simulink model "power_hvdc12_fault"  (R2016a)
settings: Solver=FixedStepDiscrete  SolverMode=SingleTasking  StartTime=0.0  StopTime=2  FixedStep=Ts  RelTol=1e-3  AbsTol=1e-2
InitFcn:
  | Ts=50e-6;
  | 
  | % Rectifier AC side :
  | VLL_nom_R = 500e3; % V
  | Fnom_R = 60;           % Hz
  | 
  | % Inverter AC side :
  | VLL_nom_I = 345e3; % V
  | Fnom_I = 50;           % Hz
  | 
  | % DC :
  | Vdc_nom = 500e3;   % V
  | Idc_nom  = 2000;     % A
values from neighbouring files (symbols this model uses):
  m = mrand(i)    [01_Generate_TrainData_script.m]    (also in 05_Generate_TestData_script.m)
  MyTs = 1.0e-4    (= 0.0001)    [01_Generate_TrainData_script.m]    (also in 05_Generate_TestData_script.m)
undefined symbols (not defined in the file or in its folder): D1, Delta, lagging, pulse, test_alpha
libraries: powerlib_meascontrol x57, powerlib x43, simulink x24
(part 2 of 5)

== system power_hvdc12_fault/Inverter Control and Protection/Gamma Measurement ==
  Vabc : Inport
  I_th(1-6)_Y : Inport  Port=2
  I_th(1-6)_D : Inport  Port=3
  Freq : Inport  Port=4
  PulsesY : Inport  Port=5
  PulsesD : Inport  Port=6
  A--> pu : Gain  Gain=1/Idc_nom  SaturateOnIntegerOverflow=on  OutDataTypeStr=Inherit: Same as input  ParamDataTypeStr=Inherit: Same as input
  "A--> pu " : Gain  Gain=1/Idc_nom  SaturateOnIntegerOverflow=on  OutDataTypeStr=Inherit: Same as input  ParamDataTypeStr=Inherit: Same as input
  Gamma Measurement (D1 bridge) : Subsystem  DialogController=POWERSYS.PowerSysDialog  mask(Discrete Gamma Measurement (6-pulse converter)){transfo_type=Yg / D1(lag), f0=Fnom_I, Ith_min=0.001, Interpolation=on, V_tol=0.01, Ts=Ts}
      mask prompts: transfo_type "Transformer connection:"; f0 "Base frequency (Hz):"; Ith_min "Current threshold for thyristor zero-current detection (pu or A):"; Interpolation "Use interpolation"; V_tol "Voltage threshold for linear interpolation  (pu or V):"; Ts "Sample time (s):"
      mask help:
      | This block measures the extinction angle Gamma of a 6-pulse thyristor converter.
      |
      | Press Help for details.
      mask init:
      | powericon('psbcallbacks',gcb,'Discrete Gamma Measurement');
      | power_initmask();
      | if strcmp(Interpolation,'on')
      |     InterpolationOn=1;
      | else
      |     InterpolationOn=0;
      | end
      mask Help:
      | This block measures the extinction angle Gamma for each of the 6 thyristors
      | of a 6-pulse thyristor converter.
      | 
      | Gamma is the time expressed in degrees from the thyristor normal current
      | extinction to the time when the thyristor commutation voltage Vak becomes
      | positive. If interpolation is activated, Gamma is evaluated more precisely
      | by predicting the "exact" zero crossing instant of commutation voltage.
      | Interpolation is applied only if the voltage variation between the two
      | voltage samples on each side of zero-crossing exceeds the value specified
      | in the "Voltage threshold for interpolation" parameter (recommended value
      | 1% of nominal voltage).
      | 
      | The system frequency (input 3) is used to convert time values in electrical
      |  degrees. The current extinction time is determined from the "Current
      | threshold" parameter (recommended value 0.1% of nominal current). Valve
      | gate pulses (input 4) are used to discriminate between a current extinction
      |  during normal commutation sequence (valve gate pulse no longer present)
      | and premature extinction due to current discontinuity when DC current
      | reference Id_ref is low, (typically Id_ref<0.1 pu). If gate pulses are not
      | connected to input 4, Gamma measurement will stay correct as long as there
      | is no discontinuity in valve current pulses.
      | 
      | The 6 Gamma angles are determined using the 6 thyristor currents (input 1)
      | and the 6 commutation voltages derived from the three phase-to-ground AC
      | voltages measured at the primary of the converter transformer (input 2).
      | The secondary winding connection of the converter transformer (Y or Delta)
      | is selectable from the "Transformer connection" parameter. This information
      |  is important to derive the correct commutation voltage, for the outgoing
      | valve, from the primary voltages.
      | 
      | Output 1 = minimum value of the 6 Gamma angles over a rolling window of 6
      | consecutive extinctions; Output 2= mean value of the 6 Gamma angles; Output
      |  3 = vector of 6 commutation voltages used in the determination of Gamma,
      | assuming a 1:1 converter transformer ratio; Output 4= scalar output of the
      | six gamma angles.
      mask TypeOptions transfo_type: Yg / Y | Yg / D1(lag) | Yg / D11(lead)
      mask Callback Interpolation: powericon('psbcallbacks',gcb,'Discrete Gamma Measurement');
      mask Display: disp('\n\n\n')
  Gamma Measurement (Y bridge) : Subsystem  DialogController=POWERSYS.PowerSysDialog  mask(Discrete Gamma Measurement (6-pulse converter)){transfo_type=Yg / Y, f0=Fnom_I, Ith_min=0.001, Interpolation=on, V_tol=0.01, Ts=Ts}
      mask prompts: transfo_type "Transformer connection:"; f0 "Base frequency (Hz):"; Ith_min "Current threshold for thyristor zero-current detection (pu or A):"; Interpolation "Use interpolation"; V_tol "Voltage threshold for linear interpolation  (pu or V):"; Ts "Sample time (s):"
      mask help:
      | This block measures the extinction angle Gamma of a 6-pulse thyristor converter.
      |
      | Press Help for details.
      mask init:
      | powericon('psbcallbacks',gcb,'Discrete Gamma Measurement');
      | power_initmask();
      | if strcmp(Interpolation,'on')
      |     InterpolationOn=1;
      | else
      |     InterpolationOn=0;
      | end
      mask Help:
      | This block measures the extinction angle Gamma for each of the 6 thyristors
      | of a 6-pulse thyristor converter.
      | 
      | Gamma is the time expressed in degrees from the thyristor normal current
      | extinction to the time when the thyristor commutation voltage Vak becomes
      | positive. If interpolation is activated, Gamma is evaluated more precisely
      | by predicting the "exact" zero crossing instant of commutation voltage.
      | Interpolation is applied only if the voltage variation between the two
      | voltage samples on each side of zero-crossing exceeds the value specified
      | in the "Voltage threshold for interpolation" parameter (recommended value
      | 1% of nominal voltage).
      | 
      | The system frequency (input 3) is used to convert time values in electrical
      |  degrees. The current extinction time is determined from the "Current
      | threshold" parameter (recommended value 0.1% of nominal current). Valve
      | gate pulses (input 4) are used to discriminate between a current extinction
      |  during normal commutation sequence (valve gate pulse no longer present)
      | and premature extinction due to current discontinuity when DC current
      | reference Id_ref is low, (typically Id_ref<0.1 pu). If gate pulses are not
      | connected to input 4, Gamma measurement will stay correct as long as there
      | is no discontinuity in valve current pulses.
      | 
      | The 6 Gamma angles are determined using the 6 thyristor currents (input 1)
      | and the 6 commutation voltages derived from the three phase-to-ground AC
      | voltages measured at the primary of the converter transformer (input 2).
      | The secondary winding connection of the converter transformer (Y or Delta)
      | is selectable from the "Transformer connection" parameter. This information
      |  is important to derive the correct commutation voltage, for the outgoing
      | valve, from the primary voltages.
      | 
      | Output 1 = minimum value of the 6 Gamma angles over a rolling window of 6
      | consecutive extinctions; Output 2= mean value of the 6 Gamma angles; Output
      |  3 = vector of 6 commutation voltages used in the determination of Gamma,
      | assuming a 1:1 converter transformer ratio; Output 4= scalar output of the
      | six gamma angles.
      mask TypeOptions transfo_type: Yg / Y | Yg / D1(lag) | Yg / D11(lead)
      mask Callback Interpolation: powericon('psbcallbacks',gcb,'Discrete Gamma Measurement');
      mask Display: disp('\n\n\n')
  MinMax1 : MinMax  Inputs=2  SaturateOnIntegerOverflow=on  InputSameDT=on
  Selector : Selector  InputPortWidth=6  IndexOptions=Index vector (dialog)  Indices=1  OutputSizes=1
  Selector1 : Selector  InputPortWidth=6  IndexOptions=Index vector (dialog)  Indices=1  OutputSizes=1
  Sum1 : Sum  SaturateOnIntegerOverflow=on  InputSameDT=on  OutDataTypeStr=Inherit: Same as first input
  Terminator1 : Terminator
  Terminator2 : Terminator
  Terminator3 : Terminator
  k : Gain  Gain=0.5  SaturateOnIntegerOverflow=on  OutDataTypeStr=Inherit: Same as input  ParamDataTypeStr=Inherit: Same as input
  gamma_min : Outport
  gamma_mean : Outport  Port=2
  tag scope: ISw1Y_pu=global, Ucom1Y_pu=global
  wires:
  I_th(1-6)_Y/1 -> A--> pu/1
  A--> pu/1 -> Gamma Measurement (Y bridge)/1(I_th(1-6)), Selector1/1
  Vabc/1 -> Gamma Measurement (D1 bridge)/2(Uabc), Gamma Measurement (Y bridge)/2(Uabc)
  Gamma Measurement (Y bridge)/1(gamma_min (deg)) -> MinMax1/1  "gamma min Y"
  Gamma Measurement (Y bridge)/3(Ucom(1-6)) -> Selector/1
  Gamma Measurement (Y bridge)/2(gamma_mean (deg)) -> Sum1/1
  I_th(1-6)_D/1 -> "A--> pu "/1
  "A--> pu "/1 -> Gamma Measurement (D1 bridge)/1(I_th(1-6))
  Gamma Measurement (D1 bridge)/3(Ucom(1-6)) -> Terminator2/1
  Gamma Measurement (D1 bridge)/2(gamma_mean (deg)) -> Sum1/2
  Gamma Measurement (D1 bridge)/1(gamma_min (deg)) -> MinMax1/2  "gamma min D"
  MinMax1/1 -> gamma_min/1
  Sum1/1 -> k/1
  k/1 -> gamma_mean/1
  Selector/1 -> [Ucom1Y_pu]
  Selector1/1 -> [ISw1Y_pu]
  Freq/1 -> Gamma Measurement (D1 bridge)/3(Freq), Gamma Measurement (Y bridge)/3(Freq)
  Gamma Measurement (D1 bridge)/4(gamma (deg)) -> Terminator1/1
  Gamma Measurement (Y bridge)/4(gamma (deg)) -> Terminator3/1
  PulsesY/1 -> Gamma Measurement (Y bridge)/4(Pulses(1-6))
  PulsesD/1 -> Gamma Measurement (D1 bridge)/4(Pulses(1-6))

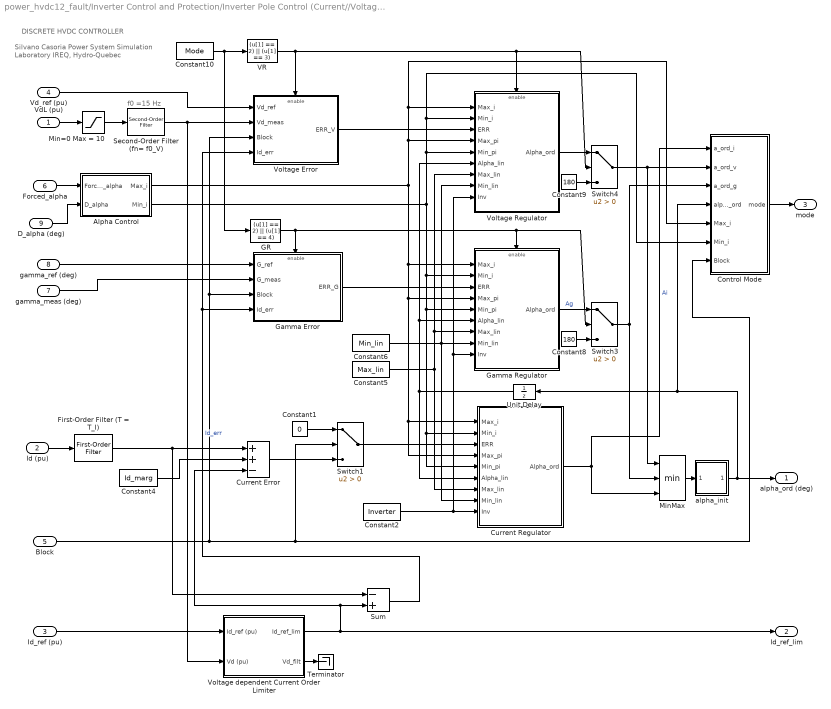
== system power_hvdc12_fault/Inverter Control and Protection/Inverter Pole Control (Current//Voltage//Gamma) ==
  note: DISCRETE HVDC CONTROLLER
  note: Silvano Casoria
      | Power System Simulation Laboratory
      |  IREQ, Hydro-Quebec
  note: f0 =15 Hz
  VdL (pu) : Inport
  Id (pu) : Inport  Port=2
  Id_ref (pu) : Inport  Port=3
  Vd_ref (pu) : Inport  Port=4
  Block : Inport  Port=5
  Forced_alpha : Inport  Port=6
  gamma_meas (deg) : Inport  Port=7
  gamma_ref (deg) : Inport  Port=8
  D_alpha (deg) : Inport  Port=9
  Alpha Control : Subsystem
  Constant1 : Constant  Value=0
  Constant10 : Constant  Value=Mode
  Constant2 : Constant  Value=Inverter
  Constant4 : Constant  Value=Id_marg
  Constant5 : Constant  Value=Max_lin
  Constant6 : Constant  Value=Min_lin
  Constant8 : Constant  Value=180
  Constant9 : Constant  Value=180
  "Control Mode " : Subsystem
  Current Error : Sum  Inputs=++-  SaturateOnIntegerOverflow=on  InputSameDT=on  OutDataTypeStr=Inherit: Same as first input
  Current Regulator : Subsystem  TreatAsAtomicUnit=on
  First-Order Filter (T = T_I) : powerlib_meascontrol/Filters/First-Order Filter  FilterType=Lowpass  Tc=T_I  Ts=Ts  Initialize=off  Vac_Init=[0, 0, 60]  Vdc_Init=0  PlotResponse=off  FreqRange="[0,  200,  1]"
  GR : Fcn  Expr=(u[1] == 2) || (u[1] == 4)
  Gamma Error : Subsystem  TreatAsAtomicUnit=on
  Gamma Regulator : Subsystem  TreatAsAtomicUnit=on
  Min=0 Max = 10 : Saturate  UpperLimit=10  LowerLimit=0
  MinMax : MinMax  Inputs=3  SaturateOnIntegerOverflow=on  InputSameDT=on
  Second-Order Filter (fn= f0_V) : powerlib_meascontrol/Filters/Second-Order Filter  FilterType=Lowpass  Fo=f0_V  Zeta=Z_V  Ts=Ts  Initialize=off  Vac_Init="[0,  0,  60]"  Vdc_Init=0  PlotResponse=off  FreqRange=[0, 500, 1]
  Sum : Sum  Inputs=-+  SaturateOnIntegerOverflow=on  InputSameDT=on  OutDataTypeStr=Inherit: Same as first input
  Switch1 : Switch  Criteria=u2 > Threshold  SaturateOnIntegerOverflow=on  InputSameDT=on
  Switch3 : Switch  Criteria=u2 > Threshold  SaturateOnIntegerOverflow=on  InputSameDT=on
  Switch4 : Switch  Criteria=u2 > Threshold  SaturateOnIntegerOverflow=on  InputSameDT=on
  Terminator : Terminator
  Unit Delay : UnitDelay  SampleTime=Ts
  VR : Fcn  Expr=(u[1] == 2) || (u[1] == 3)
  Voltage Error : Subsystem  TreatAsAtomicUnit=on
  Voltage Regulator : Subsystem  TreatAsAtomicUnit=on
  Voltage dependent Current Order Limiter : Subsystem  mask(Voltage Dependent Current Order Limiter  (Discrete)){Vd_seuil=Vd_seuil, Vd_min=Vd_min, Id_min=Id_min, Id_min_abs=Id_min_abs, Tu=Tup, Ts=Ts}
      mask prompts: Vd_seuil "Vd seuil (pu):"; Vd_min "Vd min (pu):"; Id_min "Id min (pu):"; Id_min_abs "Id min abs (pu):"; Tu "Up Time constant (s):"; Ts "Sample time (s):"
      mask Display: disp('VDCOL\n (Discrete)')
  alpha_init : Subsystem
  alpha_ord (deg) : Outport
  Id_ref_lim : Outport  Port=2
  mode : Outport  Port=3
  wires:
  Voltage Regulator/1(Alpha_ord) -> Switch4/1
  GR/1 -> Gamma Error/Enable, Gamma Regulator/Enable, Switch3/2
  Constant10/1 -> VR/1, GR/1
  VR/1 -> Voltage Error/Enable, Switch4/2, Voltage Regulator/Enable
  D_alpha (deg)/1 -> Alpha Control/2(D_alpha)
  Alpha Control/1(Max_i) -> Current Regulator/1(Max_i), Current Regulator/4(Max_pi), Gamma Regulator/4(Max_pi), Gamma Regulator/1(Max_i), "Control Mode "/5(Max_i), Voltage Regulator/1(Max_i), Voltage Regulator/4(Max_pi)
  Constant6/1 -> Voltage Regulator/8(Min_lin), Gamma Regulator/8(Min_lin), Current Regulator/8(Min_lin)
  Constant4/1 -> Current Error/2
  Id_ref (pu)/1 -> Voltage dependent Current Order Limiter/1(Id_ref (pu))
  Voltage dependent Current Order Limiter/2(Vd_filt) -> Terminator/1
  Voltage dependent Current Order Limiter/1(Id_ref_lim) -> Id_ref_lim/1, Sum/2, Current Error/3
  Second-Order Filter (fn= f0_V)/1 -> Voltage dependent Current Order Limiter/2(Vd (pu)), Voltage Error/2(Vd_meas)
  Min=0 Max = 10/1 -> Second-Order Filter (fn= f0_V)/1
  VdL (pu)/1 -> Min=0 Max = 10/1
  Id (pu)/1 -> First-Order Filter (T = T_I)/1
  First-Order Filter (T = T_I)/1 -> Sum/1, Current Error/1
  Current Error/1 -> Switch1/3
  MinMax/1 -> alpha_init/1(In1)
  Unit Delay/1 -> Voltage Regulator/6(Alpha_lin), Gamma Regulator/6(Alpha_lin), Current Regulator/6(Alpha_lin)
  alpha_init/1(Out1) -> alpha_ord (deg)/1, Unit Delay/1, "Control Mode "/4(alpha_ord)
  Constant5/1 -> Voltage Regulator/7(Max_lin), Gamma Regulator/7(Max_lin), Current Regulator/7(Max_lin)
  Alpha Control/2(Min_i) -> Current Regulator/5(Min_pi), Current Regulator/2(Min_i), Gamma Regulator/5(Min_pi), Gamma Regulator/2(Min_i), "Control Mode "/6(Min_i), Voltage Regulator/2(Min_i), Voltage Regulator/5(Min_pi)
  Block/1 -> Switch1/2, "Control Mode "/7(Block), Gamma Error/3(Block), Voltage Error/3(Block)
  Constant2/1 -> Voltage Regulator/9(Inv), Gamma Regulator/9(Inv), Current Regulator/9(Inv)
  Switch1/1 -> Current Regulator/3(ERR)
  Gamma Regulator/1(Alpha_ord) -> Switch3/1  "Ag"
  Constant8/1 -> Switch3/3
  Constant9/1 -> Switch4/3
  Current Regulator/1(Alpha_ord) -> MinMax/3, "Control Mode "/1("a_ord_i ")  "Ai"
  Switch3/1 -> MinMax/2, "Control Mode "/3(a_ord_g)
  Switch4/1 -> MinMax/1, "Control Mode "/2(a_ord_v)
  Constant1/1 -> Switch1/1
  Gamma Error/1(ERR_G) -> Gamma Regulator/3(ERR)
  gamma_ref (deg)/1 -> Gamma Error/1(G_ref)
  gamma_meas (deg)/1 -> Gamma Error/2(G_meas)
  Sum/1 -> Voltage Error/4(Id_err), Gamma Error/4(Id_err)  "Id_err"
  Vd_ref (pu)/1 -> Voltage Error/1(Vd_ref)
  Voltage Error/1(ERR_V) -> Voltage Regulator/3(ERR)
  "Control Mode "/1(mode) -> mode/1
  Forced_alpha/1 -> Alpha Control/1(Forced_alpha)

== system power_hvdc12_fault/Inverter Control and Protection/Inverter Protections ==
  Uabc (pu) : Inport
  Commutation Failure Prevention Control (CFPREV) : Subsystem  mask(Commutation Failure Prevention Control){STATE=on, T_ss=0.64, ab_level=0.1, ab_gain=25, z_level=0.1, z_gain=25, fn=60, Filter=[2.0, 1.0], Ts=Ts}
      mask prompts: STATE "ON State"; T_ss "Simulation Steady_State Time (s):"; ab_level "ab level (pu):"; ab_gain "ab gain (deg/pu):"; z_level "z level (pu):"; z_gain "z gain (deg/pu):"; fn "Base frequency (Hz):"; Filter "Filter Time const. and Iinitial condition [T(s), Ic (pu)]:"; Ts "Sample Time (s):"
      mask help:
      | The protective function, used in the inverter, mitigates commutation failures due to AC voltage dips. After a fault detection (three-phase or one-phase) an angle value (AMIN_CFPREV) is sent to the converter control in order to be deducted from the maximum delay angle limit (alpha_max). Practically, the commutation margin is consequently enlarged reducing therefore the risk of commutation failures.
      |
      |      The CLARK transformation is used for three-phase fault  detection and the zero-sequence voltage evaluation. The detection is based  on instantaneous values, which ensure fast reaction of the control system when AC faults occurs.
      |
      |      Press Help to get the reference with the  detailed description of the function and  parameters.
      |
      | Note: To accelerate the function initialisation, the first parameter (Simulation Steady_State Time) is used. It corresponds to the time when the input voltages reache  the steady-state value.
      mask init:
      | T_periode = 0.6/fn;    % More then half the period
      | filt_tc = Filter(1);
      | filt_ic = Filter(2);
      | 
      | if (STATE)
      | 	str = 'ON';
      | else
      | 	str = 'OFF';
      | end
      mask Help:
      | Ref. "A Novel Method to Mitigate Commutation Failures in HVDC Systems,"
      | Lidong Zhang, Lars Dofnas ABB Utilities Power System Technology,
      | Proceedings PowerCon 2002, Volume: 1 , 13-17 Oct. 2002,  Page(s): 51-56 vol.1.
      mask Display: disp(['\n\n\n State:[',str,']'])
  First-Order Filter (T= 3.3 ms) : powerlib_meascontrol/Filters/First-Order Filter  FilterType=Lowpass  Tc=0.0033  Ts=Ts  Initialize=off  Vac_Init=[0, 0, 60]  Vdc_Init=0  PlotResponse=off  FreqRange="[0,  200,  1]"
  Informations : Subsystem
      mask Display: disp('?')
  Low  AC Voltage Detection (LACVD) : Subsystem  TreatAsAtomicUnit=on  mask(Low AC voltage detection){STATE=on, Ref_1=0.75, Ts=fix(0.001/Ts)*Ts}
      mask prompts: STATE "ON State"; Ref_1 "Detection level (pu):"; Ts "Sample time (s):"
      mask help:
      | This bloc detects a low AC voltage condition on the commutation busbar and is used in the DC protection scheme. Its purpose is to descriminate between a drop in the AC voltage caused by a fault on the DC line or by a fault on the AC side.
      |
      |      An AC fault detection (Low_ac_voltage output signal) will occur when the AC voltage input (recified three-phase AC voltage) drops below a certain reference value (Detection level).
      |
      |      In order to minimize the simulation time, an enabled susbystem having a sample time of 1 (ms) has been used in accordance with an acceptable precision.
      mask init:
      | if (STATE)
      | 	str = 'ON';
      | else
      | 	str = 'OFF';
      | end
      mask Display: disp(['\n\n\n\nState:[',str,']'])
  T = 1 ms : DiscretePulseGenerator  Period=fix(0.001/Ts)  SampleTime=Ts
  Udio_6p : Subsystem
  Low_AC_Voltage : Outport
  AMIN_CFPREV : Outport  Port=2
  wires:
  Uabc (pu)/1 -> Udio_6p/1(Uabc (pu)), Commutation Failure Prevention Control (CFPREV)/1(Uabc (pu))
  Low  AC Voltage Detection (LACVD)/1(Low_AC_Voltage) -> Low_AC_Voltage/1
  Commutation Failure Prevention Control (CFPREV)/1(AMIN_CFPREV (deg)) -> AMIN_CFPREV/1
  T = 1 ms/1 -> Low  AC Voltage Detection (LACVD)/Enable
  Udio_6p/1(Udio_6p) -> First-Order Filter (T= 3.3 ms)/1
  First-Order Filter (T= 3.3 ms)/1 -> Low  AC Voltage Detection (LACVD)/1(Uac (pu))

== system power_hvdc12_fault/Master Control/Informations ==
  note: For testing purpose,  a step can be activated and added to the reference current at both
      | converters.
  note: Master Control
  note: INTRODUCTION
  note: The rectifier and inverter current reference are generated in the master control. The reference
      | should be equal in both converters to avoid the loss of the margin. The converter starting and stopping is
      | initiated and the current reference can be ramped up or down.  A current step can be added to the
      | current reference for testing purpose.
  note: DESCRIPTION
  note: At start-up, both converters are deblocked and ramped up to the minimum current allowed in steady-state
      | with an adjustable rate  and application time in the "Start/Stop & Ramping Unit" subsystem. After the
      | system stabilisation the current is ramped up to its final value  with an adjustable rate and execution time.
      | Before stopping the converters the current is ramped down to the minimum reference.

== system power_hvdc12_fault/Master Control/Start//Stop ==
  note: Start/Stop sequence
  note: Start/Stop & Ramping
  note: Ramping
  Bistable : powerlib_meascontrol/Logic/Bistable  Qpriority=Set  ic=0  Ts=Ts
  Edge Detector_1 : powerlib_meascontrol/Logic/Edge Detector  model=Rising  ic=0  Ts=Ts
  Edge Detector_2 : powerlib_meascontrol/Logic/Edge Detector  model=Rising  ic=0  Ts=Ts
  Logical Operator3 : Logic  AllPortsSameDT=off
  Minimum ref : Constant  Value=Min_ref
  Relational Operator1 : RelationalOperator  Operator=<=
  S1 : Subsystem  mask(RAMPING UNIT){Min_ref=Min_ref, SS_ramp=SS_ramp, F_up=F_up, up_slope=up_slope, T_up=T_up, F_down=F_down, down_slope=down_slope, T_down=T_down}
      mask prompts: Min_ref "Minimum Value (pu):"; SS_ramp "Start-Stop ramp (pu/s):"; F_up "Final Up Value (pu):"; up_slope "Up Slope (pu/s):"; T_up "Ramping Up Time (s):"; F_down "Final Down Value (pu):"; down_slope "Down Slope (pu/s):"; T_down "Ramping Down Time (s):"
      mask init:
      | T_up_final      =  T_up + (F_up - Min_ref)/up_slope;
      | T_down_final =   T_down + (F_down-F_up)/down_slope;
      | T_ramp  = [0, T_up, T_up_final,  T_down,  T_down_final, 9999]';
      | U_ramp = [0, 0, F_up-Min_ref,  F_up-Min_ref,  F_down- Min_ref,  F_down - Min_ref]';
      mask Display: disp('Ramping\n Unit')
  Start (T_start) : Step  Time=T_start  SampleTime=Ts
  Stop (T_stop) : Step  Time=T_stop  SampleTime=Ts
  Unit Delay : UnitDelay  SampleTime=Ts
  Id_ref_ramp : Outport
  "Stop " : Outport  Port=2
  wires:
  S1/1(Out1) -> Unit Delay/1, Id_ref_ramp/1
  Minimum ref/1 -> Relational Operator1/2
  Unit Delay/1 -> Relational Operator1/1
  Start (T_start)/1 -> Edge Detector_1/1
  Bistable/1 -> S1/1(Start)  "Start"
  Relational Operator1/1 -> Logical Operator3/1
  Stop (T_stop)/1 -> Logical Operator3/2
  Logical Operator3/1 -> Edge Detector_2/1
  Bistable/2 -> "Stop "/1
  Edge Detector_1/1 -> Bistable/1
  Edge Detector_2/1 -> Bistable/2

== system power_hvdc12_fault/Rectifier/Rectifier ==
  Py : Inport
  Pd : Inport  Port=2
  Bridge D : powerlib/Power Electronics/Universal Bridge  Arms=3  SnubberResistance=2000  SnubberCapacitance=0.1e-6  Device=Thyristors  Ron=1e-3  Lon=0  ForwardVoltages="[  0.8  0.8  ]"  ForwardVoltage=0  GTOparameters=[ 10e-6 , 20e-6 ]  IGBTparameters=[ 1e-6 , 2e-6 ]  Measurements=None  Measurements_2=None  converterType=Rectifier
  Bridge Y : powerlib/Power Electronics/Universal Bridge  Arms=3  SnubberResistance=2000  SnubberCapacitance=0.1e-6  Device=Thyristors  Ron=1e-3  Lon=0  ForwardVoltages="[  0.8  0.8  ]"  ForwardVoltage=0  GTOparameters=[ 10e-6 , 20e-6 ]  IGBTparameters=[ 1e-6 , 2e-6 ]  Measurements=All voltages and currents  Measurements_2=None  converterType=Rectifier
  Ay : PMIOPort  Port=1  Side=Left
  By : PMIOPort  Port=2  Side=Left
  Cy : PMIOPort  Port=3  Side=Left
  Ad : PMIOPort  Port=4  Side=Left
  Bd : PMIOPort  Port=5  Side=Left
  Cd : PMIOPort  Port=6  Side=Left
  pos : PMIOPort  Port=7  Side=Right
  neg : PMIOPort  Port=8  Side=Right
  wires:
  Pd/1 -> Bridge D/1
  Py/1 -> Bridge Y/1
  connections:
  Bridge D/RConn2 -- neg/RConn1
  Cd/RConn1 -- Bridge D/LConn3
  Bd/RConn1 -- Bridge D/LConn2
  Ad/RConn1 -- Bridge D/LConn1
  Cy/RConn1 -- Bridge Y/LConn3
  By/RConn1 -- Bridge Y/LConn2
  Bridge Y/RConn1 -- pos/RConn1
  Ay/RConn1 -- Bridge Y/LConn1
  Bridge D/RConn1 -- Bridge Y/RConn2

== system power_hvdc12_fault/Rectifier Control and Protection/12-pulse Firing Control ==
  alpha_ord (deg) : Inport
  Vabc (pu) : Inport  Port=2
  Block : Inport  Port=3
  PLL (3ph) : powerlib_meascontrol/PLL/PLL (3ph)  Fmin=0.75 * PLL_f0  Par_Init="[PLL_ph  PLL_f0]"  ParK="[PLL_Kp  PLL_Ki  0]"  TcD=1e-4  MaxRateChangeFreq=12  FilterCutOffFreq=25  Ts=Ts  AGC=off
  "Pulse Generator (Thyristor, 12-Pulse)" : powerlib_meascontrol/Pulse & Signal Generators/Pulse Generator (Thyristor, 12-Pulse)  GenType=12-pulse  Delta=D1 (lagging)  pwidth=Pw  Double_Pulse=off  Ts=Ts
  PulsesY : Outport
  PulsesD : Outport  Port=2
  Freq : Outport  Port=3
  wires:
  Vabc (pu)/1 -> PLL (3ph)/1
  PLL (3ph)/2 -> "Pulse Generator (Thyristor, 12-Pulse)"/2
  alpha_ord (deg)/1 -> "Pulse Generator (Thyristor, 12-Pulse)"/1
  "Pulse Generator (Thyristor, 12-Pulse)"/1 -> PulsesY/1
  "Pulse Generator (Thyristor, 12-Pulse)"/2 -> PulsesD/1
  PLL (3ph)/1 -> Freq/1
  Block/1 -> "Pulse Generator (Thyristor, 12-Pulse)"/3

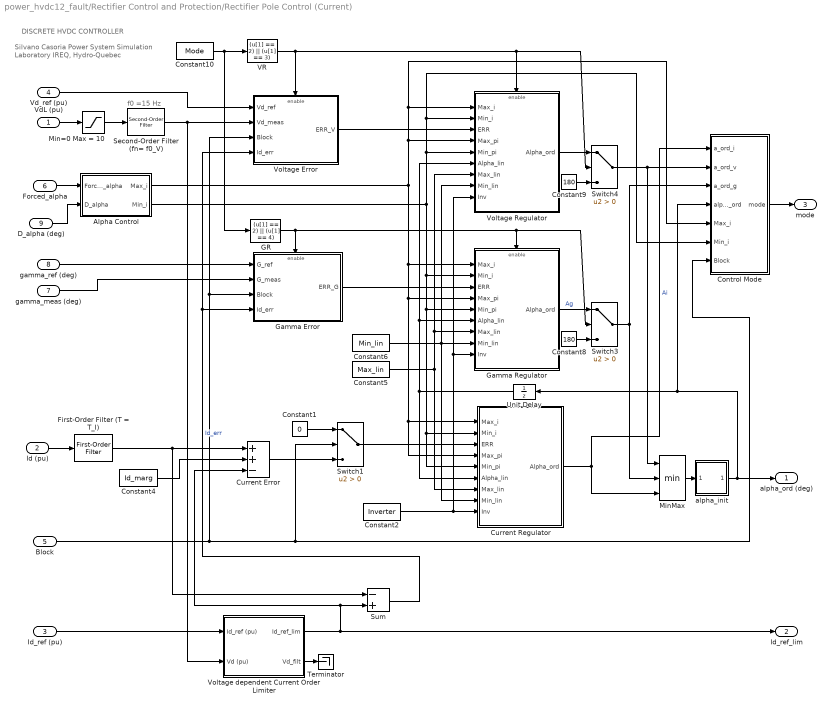
== system power_hvdc12_fault/Rectifier Control and Protection/Rectifier Pole Control (Current) ==
  note: DISCRETE HVDC CONTROLLER
  note: Silvano Casoria
      | Power System Simulation Laboratory
      |  IREQ, Hydro-Quebec
  note: f0 =15 Hz
  VdL (pu) : Inport
  Id (pu) : Inport  Port=2
  Id_ref (pu) : Inport  Port=3
  Vd_ref (pu) : Inport  Port=4
  Block : Inport  Port=5
  Forced_alpha : Inport  Port=6
  gamma_meas (deg) : Inport  Port=7
  gamma_ref (deg) : Inport  Port=8
  D_alpha (deg) : Inport  Port=9
  Alpha Control : Subsystem
  Constant1 : Constant  Value=0
  Constant10 : Constant  Value=Mode
  Constant2 : Constant  Value=Inverter
  Constant4 : Constant  Value=Id_marg
  Constant5 : Constant  Value=Max_lin
  Constant6 : Constant  Value=Min_lin
  Constant8 : Constant  Value=180
  Constant9 : Constant  Value=180
  "Control Mode " : Subsystem
  Current Error : Sum  Inputs=++-  SaturateOnIntegerOverflow=on  InputSameDT=on  OutDataTypeStr=Inherit: Same as first input
  Current Regulator : Subsystem  TreatAsAtomicUnit=on
  First-Order Filter (T = T_I) : powerlib_meascontrol/Filters/First-Order Filter  FilterType=Lowpass  Tc=T_I  Ts=Ts  Initialize=off  Vac_Init=[0, 0, 60]  Vdc_Init=0  PlotResponse=off  FreqRange="[0,  200,  1]"
  GR : Fcn  Expr=(u[1] == 2) || (u[1] == 4)
  Gamma Error : Subsystem  TreatAsAtomicUnit=on
  Gamma Regulator : Subsystem  TreatAsAtomicUnit=on
  Min=0 Max = 10 : Saturate  UpperLimit=10  LowerLimit=0
  MinMax : MinMax  Inputs=3  SaturateOnIntegerOverflow=on  InputSameDT=on
  Second-Order Filter (fn= f0_V) : powerlib_meascontrol/Filters/Second-Order Filter  FilterType=Lowpass  Fo=f0_V  Zeta=Z_V  Ts=Ts  Initialize=off  Vac_Init="[0,  0,  60]"  Vdc_Init=0  PlotResponse=off  FreqRange=[0, 500, 1]
  Sum : Sum  Inputs=-+  SaturateOnIntegerOverflow=on  InputSameDT=on  OutDataTypeStr=Inherit: Same as first input
  Switch1 : Switch  Criteria=u2 > Threshold  SaturateOnIntegerOverflow=on  InputSameDT=on
  Switch3 : Switch  Criteria=u2 > Threshold  SaturateOnIntegerOverflow=on  InputSameDT=on
  Switch4 : Switch  Criteria=u2 > Threshold  SaturateOnIntegerOverflow=on  InputSameDT=on
  Terminator : Terminator
  Unit Delay : UnitDelay  SampleTime=Ts
  VR : Fcn  Expr=(u[1] == 2) || (u[1] == 3)
  Voltage Error : Subsystem  TreatAsAtomicUnit=on
  Voltage Regulator : Subsystem  TreatAsAtomicUnit=on
  Voltage dependent Current Order Limiter : Subsystem  mask(Voltage Dependent Current Order Limiter  (Discrete)){Vd_seuil=Vd_seuil, Vd_min=Vd_min, Id_min=Id_min, Id_min_abs=Id_min_abs, Tu=Tup, Ts=Ts}
      mask prompts: Vd_seuil "Vd seuil (pu):"; Vd_min "Vd min (pu):"; Id_min "Id min (pu):"; Id_min_abs "Id min abs (pu):"; Tu "Up Time constant (s):"; Ts "Sample time (s):"
      mask Display: disp('VDCOL\n (Discrete)')
  alpha_init : Subsystem
  alpha_ord (deg) : Outport
  Id_ref_lim : Outport  Port=2
  mode : Outport  Port=3
  wires:
  Voltage Regulator/1(Alpha_ord) -> Switch4/1
  GR/1 -> Gamma Error/Enable, Gamma Regulator/Enable, Switch3/2
  Constant10/1 -> VR/1, GR/1
  VR/1 -> Voltage Error/Enable, Switch4/2, Voltage Regulator/Enable
  D_alpha (deg)/1 -> Alpha Control/2(D_alpha)
  Alpha Control/1(Max_i) -> Current Regulator/1(Max_i), Current Regulator/4(Max_pi), Gamma Regulator/4(Max_pi), Gamma Regulator/1(Max_i), "Control Mode "/5(Max_i), Voltage Regulator/1(Max_i), Voltage Regulator/4(Max_pi)
  Constant6/1 -> Voltage Regulator/8(Min_lin), Gamma Regulator/8(Min_lin), Current Regulator/8(Min_lin)
  Constant4/1 -> Current Error/2
  Id_ref (pu)/1 -> Voltage dependent Current Order Limiter/1(Id_ref (pu))
  Voltage dependent Current Order Limiter/2(Vd_filt) -> Terminator/1
  Voltage dependent Current Order Limiter/1(Id_ref_lim) -> Id_ref_lim/1, Sum/2, Current Error/3
  Second-Order Filter (fn= f0_V)/1 -> Voltage dependent Current Order Limiter/2(Vd (pu)), Voltage Error/2(Vd_meas)
  Min=0 Max = 10/1 -> Second-Order Filter (fn= f0_V)/1
  VdL (pu)/1 -> Min=0 Max = 10/1
  Id (pu)/1 -> First-Order Filter (T = T_I)/1
  First-Order Filter (T = T_I)/1 -> Sum/1, Current Error/1
  Current Error/1 -> Switch1/3
  MinMax/1 -> alpha_init/1(In1)
  Unit Delay/1 -> Voltage Regulator/6(Alpha_lin), Gamma Regulator/6(Alpha_lin), Current Regulator/6(Alpha_lin)
  alpha_init/1(Out1) -> alpha_ord (deg)/1, Unit Delay/1, "Control Mode "/4(alpha_ord)
  Constant5/1 -> Voltage Regulator/7(Max_lin), Gamma Regulator/7(Max_lin), Current Regulator/7(Max_lin)
  Alpha Control/2(Min_i) -> Current Regulator/5(Min_pi), Current Regulator/2(Min_i), Gamma Regulator/5(Min_pi), Gamma Regulator/2(Min_i), "Control Mode "/6(Min_i), Voltage Regulator/2(Min_i), Voltage Regulator/5(Min_pi)
  Block/1 -> Switch1/2, "Control Mode "/7(Block), Gamma Error/3(Block), Voltage Error/3(Block)
  Constant2/1 -> Voltage Regulator/9(Inv), Gamma Regulator/9(Inv), Current Regulator/9(Inv)
  Switch1/1 -> Current Regulator/3(ERR)
  Gamma Regulator/1(Alpha_ord) -> Switch3/1  "Ag"
  Constant8/1 -> Switch3/3
  Constant9/1 -> Switch4/3
  Current Regulator/1(Alpha_ord) -> MinMax/3, "Control Mode "/1("a_ord_i ")  "Ai"
  Switch3/1 -> MinMax/2, "Control Mode "/3(a_ord_g)
  Switch4/1 -> MinMax/1, "Control Mode "/2(a_ord_v)
  Constant1/1 -> Switch1/1
  Gamma Error/1(ERR_G) -> Gamma Regulator/3(ERR)
  gamma_ref (deg)/1 -> Gamma Error/1(G_ref)
  gamma_meas (deg)/1 -> Gamma Error/2(G_meas)
  Sum/1 -> Voltage Error/4(Id_err), Gamma Error/4(Id_err)  "Id_err"
  Vd_ref (pu)/1 -> Voltage Error/1(Vd_ref)
  Voltage Error/1(ERR_V) -> Voltage Regulator/3(ERR)
  "Control Mode "/1(mode) -> mode/1
  Forced_alpha/1 -> Alpha Control/1(Forced_alpha)

== system power_hvdc12_fault/Rectifier Control and Protection/Rectifier Protections ==
  note: DC Protections (in Rectifier)
  Uabc (pu) : Inport
  VdL (pu) : Inport  Port=2
  Deblocked : Inport  Port=3
  Low_ac_volt_oth : Inport  Port=4
  DC Fault Protection (DCPROT) : Subsystem  mask(DC fault protection (in Rectifier)){STATE=on, Ref1=0.5, T1=0.070, T2=0.05, polarity=Positive, Ts=fix(0.002/Ts)*Ts}
      mask prompts: STATE "ON State"; Ref1 "Detection level (pu):"; T1 "Detection delay (s):"; T2 "Forced alpha duration (s):"; polarity "Voltage polarity:"; Ts "Sample time (s):"
      mask help:
      | The protection is active in the rectifier. It will detect a fault on the DC side and will force the delay angle into the inverter region in order to extinguish the fault current.
      |      The fault detection on the DC line is based on the drop in the line to ground voltage.
      |      The normal voltage polarity (+ or -) of the line is a parameter as well as the reference level (Detection level) of the fault detection.
      |      A delay time (Detection delay) is used in the detection to descriminate between a line fault and other disturbances resulting in a low DC voltage.
      |      A delay time (200 ms) is allowed, after the DC system start-up, before activating the detection logic to make sure that the normal operating DC voltage is established.
      |      Also, an external signal (Lock) generated by another protective function (e.g. Low AC voltage detection) will lock the detection for a minimum amount of time (set by an Off Delay bloc) in order to descriminate between any fault causing a low DC voltage.
      |      A detection will triger a Forced alpha during an ajustable interval (Forced alpha duration) sufficient to allow for deionization of the fault path prior to re-application of voltage.
      |
      |      In order to minimize the simulation time, an enabled susbystem having a sample time of  2 (ms) has been used in accordance with an acceptable precision.
      mask init:
      | if (polarity == 1)
      | 	sign = 1;
      | else
      | 	sign = -1;
      | end
      | 
      | if (STATE)
      | 	str = 'ON';
      | else
      | 	str = 'OFF';
      | end
      mask TypeOptions polarity: Positive | Negative
      mask Display: disp(['\n\n\n\nState:[',str,']'])
  First-Order Filter (T=3.3 ms) : powerlib_meascontrol/Filters/First-Order Filter  FilterType=Lowpass  Tc=0.0033  Ts=Ts  Initialize=off  Vac_Init=[0, 0, 60]  Vdc_Init=0  PlotResponse=off  FreqRange=[1 500 0.1]
  Informations : Subsystem
      mask Display: disp('?')
  Logical Operator6 : Logic  Operator=OR
  Low  AC Voltage Detection (LACVD) : Subsystem  TreatAsAtomicUnit=on  mask(Low AC voltage detection){STATE=on, Ref_1=0.70, Ts=fix(0.001/Ts)*Ts}
      mask prompts: STATE "ON State"; Ref_1 "Detection level (pu):"; Ts "Sample time (s):"
      mask help:
      | This bloc detects a low AC voltage condition on the commutation busbar and is used in the DC protection scheme. Its purpose is to descriminate between a drop in the AC voltage caused by a fault on the DC line or by a fault on the AC side.
      |
      |      An AC fault detection (Low_ac_voltage output signal) will occur when the AC voltage input (recified three-phase AC voltage) drops below a certain reference value (Detection level).
      |
      |      In order to minimize the simulation time, an enabled susbystem having a sample time of 1 (ms) has been used in accordance with an acceptable precision.
      mask init:
      | if (STATE)
      | 	str = 'ON';
      | else
      | 	str = 'OFF';
      | end
      mask Display: disp(['\n\n\n\nState:[',str,']'])
  T = 1 ms : DiscretePulseGenerator  Period=fix(0.001/Ts)  SampleTime=Ts
  T = 2 ms : DiscretePulseGenerator  Period=fix(0.002/Ts)  SampleTime=Ts
  Udio_6p : Subsystem
  Forced_alpha : Outport
  Low_ac_voltage : Outport  Port=2
  wires:
  T = 1 ms/1 -> Low  AC Voltage Detection (LACVD)/Enable
  Uabc (pu)/1 -> Udio_6p/1(Uabc (pu))
  Low  AC Voltage Detection (LACVD)/1(Low_AC_Voltage) -> Logical Operator6/1, Low_ac_voltage/1
  T = 2 ms/1 -> DC Fault Protection (DCPROT)/Enable
  DC Fault Protection (DCPROT)/1(Forced_alpha) -> Forced_alpha/1
  Low_ac_volt_oth/1 -> Logical Operator6/2
  Logical Operator6/1 -> DC Fault Protection (DCPROT)/3(Lock)
  VdL (pu)/1 -> DC Fault Protection (DCPROT)/1(VdL (pu))
  Deblocked/1 -> DC Fault Protection (DCPROT)/2(Deblocked)
  First-Order Filter (T=3.3 ms)/1 -> Low  AC Voltage Detection (LACVD)/1(Uac (pu))
  Udio_6p/1(Udio_6p) -> First-Order Filter (T=3.3 ms)/1

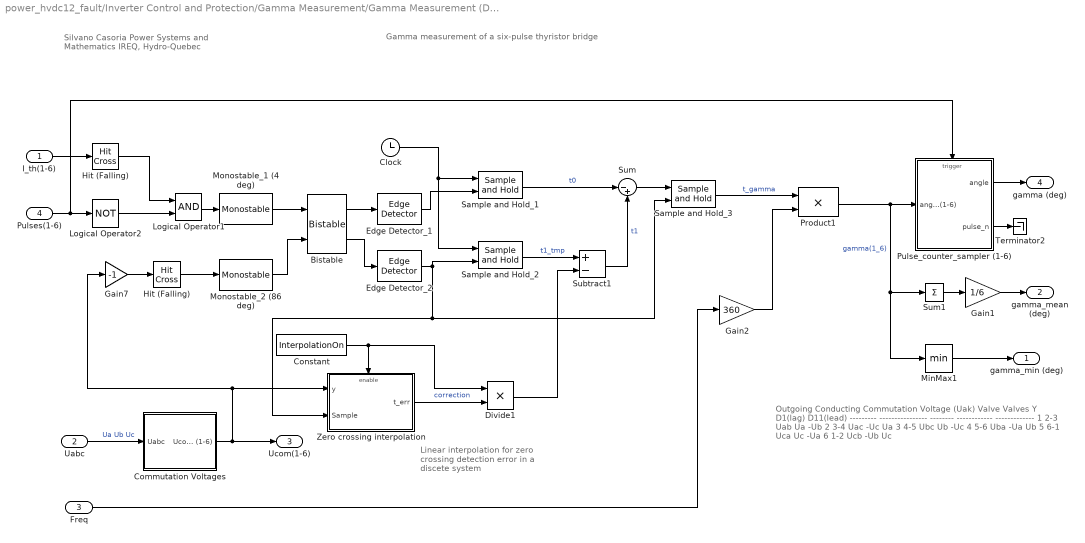
== system power_hvdc12_fault/Inverter Control and Protection/Gamma Measurement/Gamma Measurement (D1 bridge) ==
  note: Outgoing  Conducting      Commutation Voltage (Uak)
      | Valve         Valves                Y          D1(lag)     D11(lead)
      | ---------      ----------------     --------   ------------    -------------
      |     1                 2-3                Uab         Ua              -Ub
      |     2                 3-4                Uac        -Uc                Ua
      |     3                 4-5                Ubc         Ub              -Uc
      |     4                 5-6                Uba       -Ua                Ub
      |     5                 6-1                Uca         Uc              -Ua
      |     6                 1-2                Ucb        -Ub               Uc
  note: Linear interpolation for
      | zero crossing detection error
      |  in a discete system
  note: Gamma measurement of a six-pulse thyristor bridge
  note: Silvano Casoria
      | Power Systems and Mathematics
      |  IREQ, Hydro-Quebec
  I_th(1-6) : Inport  PortDimensions=6
  Uabc : Inport  Port=2  PortDimensions=3
  Freq : Inport  Port=3
  Pulses(1-6) : Inport  Port=4  PortDimensions=6
  Bistable : powerlib_meascontrol/Logic/Bistable  Qpriority=Set  ic=0  Ts=Ts
  Clock : Clock
  Commutation Voltages : Subsystem
  Constant : Constant  Value=InterpolationOn
  Divide1 : Product  Inputs=**
  Edge Detector_1 : powerlib_meascontrol/Logic/Edge Detector  model=Rising  ic=0  Ts=Ts
  Edge Detector_2 : powerlib_meascontrol/Logic/Edge Detector  model=Rising  ic=0  Ts=Ts
  Gain1 : Gain  Gain=1/6  SaturateOnIntegerOverflow=on  OutDataTypeStr=Inherit: Same as input  ParamDataTypeStr=Inherit: Same as input
  Gain2 : Gain  Gain=360  SaturateOnIntegerOverflow=on  OutDataTypeStr=Inherit: Same as input  ParamDataTypeStr=Inherit: Same as input
  Gain7 : Gain  Gain=-1  SaturateOnIntegerOverflow=on  OutDataTypeStr=Inherit: Same as input  ParamDataTypeStr=Inherit: Same as input
  Hit (Falling) : HitCross  HitCrossingOffset=Ith_min  HitCrossingDirection=falling  SampleTime=Ts
  "Hit (Falling) " : HitCross  HitCrossingDirection=falling  SampleTime=Ts
  Logical Operator1 : Logic  AllPortsSameDT=off  OutDataTypeStr=boolean
  Logical Operator2 : Logic  Operator=NOT  AllPortsSameDT=off  OutDataTypeStr=boolean
  MinMax1 : MinMax  SaturateOnIntegerOverflow=on  InputSameDT=on
  Monostable_1 (4 deg) : powerlib_meascontrol/Logic/Monostable  EdgeDetect=Rising  PulseDuration=4/(360*f0)  ic=0  Ts=Ts
  Monostable_2 (86 deg) : powerlib_meascontrol/Logic/Monostable  EdgeDetect=Rising  PulseDuration=86/(360*f0)  ic=0  Ts=Ts
  Product1 : Product  SaturateOnIntegerOverflow=on  OutDataTypeStr=Inherit: Same as first input
  Pulse_counter_sampler (1-6) : Subsystem  TreatAsAtomicUnit=on
  Sample and Hold_1 : powerlib_meascontrol/Additional Components/Sample and Hold  ic=0  Ts=Ts
  Sample and Hold_2 : powerlib_meascontrol/Additional Components/Sample and Hold  ic=0  Ts=Ts
  Sample and Hold_3 : powerlib_meascontrol/Additional Components/Sample and Hold  ic=0  Ts=Ts
  Subtract1 : Sum  Inputs=+-
  Sum : Sum  Inputs=|-+  SaturateOnIntegerOverflow=on  InputSameDT=on  OutDataTypeStr=Inherit: Same as first input
  Sum1 : Sum  Inputs=+  SaturateOnIntegerOverflow=on  InputSameDT=on  OutDataTypeStr=Inherit: Same as first input
  Terminator2 : Terminator
  Zero crossing interpolation : Subsystem  mask(Discrete - Hit crossing time interval error calculation by linear interpolation){y0=0, TOL=V_tol, Ts=Ts}
      mask prompts: y0 "Hit crossing offset (y0):"; TOL "Tolerance:"; Ts "Sample time:"
      mask help:
      | The function calculates, using the linear interpolation,an approximation of the time interval error in detencting when the input signal  (y) crosses (in any direction)the offset value "y0".
      | The output (t_err) is the time interval error which value is between 0 and the sample time. The calculation is done (otherwise t_err = 0) if the input signal changes by more then the value defined by the parameter "Tolerance".
      | This change is measured during the time step when the hit crossing takes place.
  gamma_min (deg) : Outport
  gamma_mean (deg) : Outport  Port=2
  Ucom(1-6) : Outport  Port=3
  gamma (deg) : Outport  Port=4
  wires:
  Divide1/1 -> Subtract1/2
  Pulse_counter_sampler (1-6)/2(pulse_n) -> Terminator2/1
  MinMax1/1 -> gamma_min (deg)/1
  Gain1/1 -> gamma_mean (deg)/1
  Sum1/1 -> Gain1/1
  Pulse_counter_sampler (1-6)/1(angle) -> gamma (deg)/1
  Sample and Hold_3/1 -> Product1/1  "t_gamma"
  Subtract1/1 -> Sum/2  "t1"
  Sample and Hold_1/1 -> Sum/1  "t0"
  Gain2/1 -> Product1/2
  Freq/1 -> Gain2/1
  Uabc/1 -> Commutation Voltages/1(Uabc)  "Ua Ub Uc"
  Commutation Voltages/1(Ucom (1-6)) -> Gain7/1, Zero crossing interpolation/1(y), Ucom(1-6)/1
  Gain7/1 -> "Hit (Falling) "/1
  Monostable_1 (4 deg)/1 -> Bistable/1
  "Hit (Falling) "/1 -> Monostable_2 (86 deg)/1
  Sum/1 -> Sample and Hold_3/1
  Product1/1 -> MinMax1/1, Sum1/1, Pulse_counter_sampler (1-6)/1(angles(1-6))  "gamma(1_6)"
  Edge Detector_2/1 -> Sample and Hold_2/2, Sample and Hold_3/2, Zero crossing interpolation/2(Sample)
  Pulses(1-6)/1 -> Pulse_counter_sampler (1-6)/Trigger, Logical Operator2/1
  Logical Operator2/1 -> Logical Operator1/2
  I_th(1-6)/1 -> Hit (Falling)/1
  Logical Operator1/1 -> Monostable_1 (4 deg)/1
  Hit (Falling)/1 -> Logical Operator1/1
  Constant/1 -> Zero crossing interpolation/Enable, Divide1/1
  Clock/1 -> Sample and Hold_2/1, Sample and Hold_1/1
  Zero crossing interpolation/1(t_err) -> Divide1/2  "correction"
  Bistable/1 -> Edge Detector_1/1
  Monostable_2 (86 deg)/1 -> Bistable/2
  Bistable/2 -> Edge Detector_2/1
  Edge Detector_1/1 -> Sample and Hold_1/2
  Sample and Hold_2/1 -> Subtract1/1  "t1_tmp"

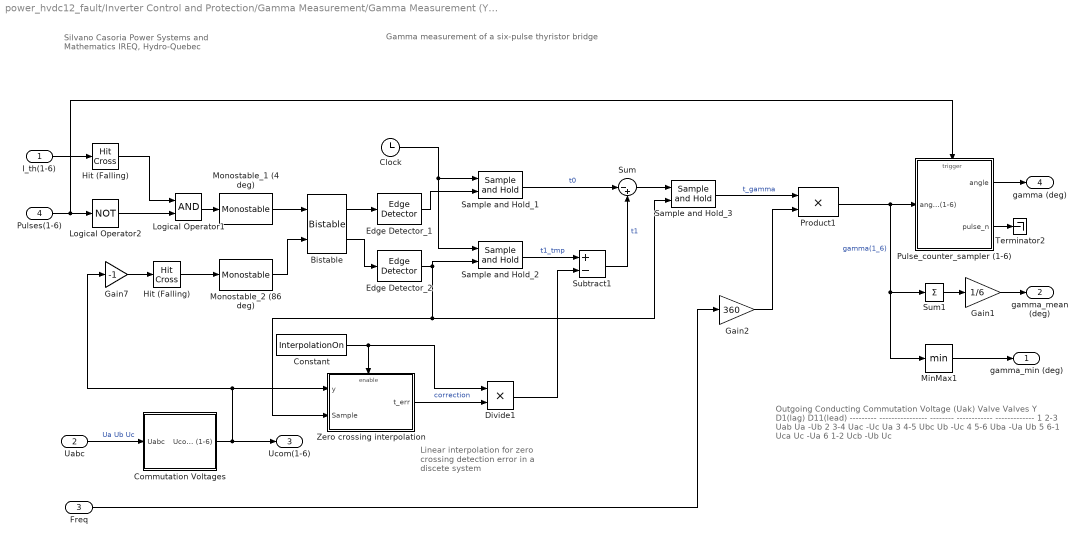
== system power_hvdc12_fault/Inverter Control and Protection/Gamma Measurement/Gamma Measurement (Y bridge) ==
  note: Outgoing  Conducting      Commutation Voltage (Uak)
      | Valve         Valves                Y          D1(lag)     D11(lead)
      | ---------      ----------------     --------   ------------    -------------
      |     1                 2-3                Uab         Ua              -Ub
      |     2                 3-4                Uac        -Uc                Ua
      |     3                 4-5                Ubc         Ub              -Uc
      |     4                 5-6                Uba       -Ua                Ub
      |     5                 6-1                Uca         Uc              -Ua
      |     6                 1-2                Ucb        -Ub               Uc
  note: Linear interpolation for
      | zero crossing detection error
      |  in a discete system
  note: Gamma measurement of a six-pulse thyristor bridge
  note: Silvano Casoria
      | Power Systems and Mathematics
      |  IREQ, Hydro-Quebec
  I_th(1-6) : Inport  PortDimensions=6
  Uabc : Inport  Port=2  PortDimensions=3
  Freq : Inport  Port=3
  Pulses(1-6) : Inport  Port=4  PortDimensions=6
  Bistable : powerlib_meascontrol/Logic/Bistable  Qpriority=Set  ic=0  Ts=Ts
  Clock : Clock
  Commutation Voltages : Subsystem
  Constant : Constant  Value=InterpolationOn
  Divide1 : Product  Inputs=**
  Edge Detector_1 : powerlib_meascontrol/Logic/Edge Detector  model=Rising  ic=0  Ts=Ts
  Edge Detector_2 : powerlib_meascontrol/Logic/Edge Detector  model=Rising  ic=0  Ts=Ts
  Gain1 : Gain  Gain=1/6  SaturateOnIntegerOverflow=on  OutDataTypeStr=Inherit: Same as input  ParamDataTypeStr=Inherit: Same as input
  Gain2 : Gain  Gain=360  SaturateOnIntegerOverflow=on  OutDataTypeStr=Inherit: Same as input  ParamDataTypeStr=Inherit: Same as input
  Gain7 : Gain  Gain=-1  SaturateOnIntegerOverflow=on  OutDataTypeStr=Inherit: Same as input  ParamDataTypeStr=Inherit: Same as input
  Hit (Falling) : HitCross  HitCrossingOffset=Ith_min  HitCrossingDirection=falling  SampleTime=Ts
  "Hit (Falling) " : HitCross  HitCrossingDirection=falling  SampleTime=Ts
  Logical Operator1 : Logic  AllPortsSameDT=off  OutDataTypeStr=boolean
  Logical Operator2 : Logic  Operator=NOT  AllPortsSameDT=off  OutDataTypeStr=boolean
  MinMax1 : MinMax  SaturateOnIntegerOverflow=on  InputSameDT=on
  Monostable_1 (4 deg) : powerlib_meascontrol/Logic/Monostable  EdgeDetect=Rising  PulseDuration=4/(360*f0)  ic=0  Ts=Ts
  Monostable_2 (86 deg) : powerlib_meascontrol/Logic/Monostable  EdgeDetect=Rising  PulseDuration=86/(360*f0)  ic=0  Ts=Ts
  Product1 : Product  SaturateOnIntegerOverflow=on  OutDataTypeStr=Inherit: Same as first input
  Pulse_counter_sampler (1-6) : Subsystem  TreatAsAtomicUnit=on
  Sample and Hold_1 : powerlib_meascontrol/Additional Components/Sample and Hold  ic=0  Ts=Ts
  Sample and Hold_2 : powerlib_meascontrol/Additional Components/Sample and Hold  ic=0  Ts=Ts
  Sample and Hold_3 : powerlib_meascontrol/Additional Components/Sample and Hold  ic=0  Ts=Ts
  Subtract1 : Sum  Inputs=+-
  Sum : Sum  Inputs=|-+  SaturateOnIntegerOverflow=on  InputSameDT=on  OutDataTypeStr=Inherit: Same as first input
  Sum1 : Sum  Inputs=+  SaturateOnIntegerOverflow=on  InputSameDT=on  OutDataTypeStr=Inherit: Same as first input
  Terminator2 : Terminator
  Zero crossing interpolation : Subsystem  mask(Discrete - Hit crossing time interval error calculation by linear interpolation){y0=0, TOL=V_tol, Ts=Ts}
      mask prompts: y0 "Hit crossing offset (y0):"; TOL "Tolerance:"; Ts "Sample time:"
      mask help:
      | The function calculates, using the linear interpolation,an approximation of the time interval error in detencting when the input signal  (y) crosses (in any direction)the offset value "y0".
      | The output (t_err) is the time interval error which value is between 0 and the sample time. The calculation is done (otherwise t_err = 0) if the input signal changes by more then the value defined by the parameter "Tolerance".
      | This change is measured during the time step when the hit crossing takes place.
  gamma_min (deg) : Outport
  gamma_mean (deg) : Outport  Port=2
  Ucom(1-6) : Outport  Port=3
  gamma (deg) : Outport  Port=4
  wires:
  Divide1/1 -> Subtract1/2
  Pulse_counter_sampler (1-6)/2(pulse_n) -> Terminator2/1
  MinMax1/1 -> gamma_min (deg)/1
  Gain1/1 -> gamma_mean (deg)/1
  Sum1/1 -> Gain1/1
  Pulse_counter_sampler (1-6)/1(angle) -> gamma (deg)/1
  Sample and Hold_3/1 -> Product1/1  "t_gamma"
  Subtract1/1 -> Sum/2  "t1"
  Sample and Hold_1/1 -> Sum/1  "t0"
  Gain2/1 -> Product1/2
  Freq/1 -> Gain2/1
  Uabc/1 -> Commutation Voltages/1(Uabc)  "Ua Ub Uc"
  Commutation Voltages/1(Ucom (1-6)) -> Gain7/1, Zero crossing interpolation/1(y), Ucom(1-6)/1
  Gain7/1 -> "Hit (Falling) "/1
  Monostable_1 (4 deg)/1 -> Bistable/1
  "Hit (Falling) "/1 -> Monostable_2 (86 deg)/1
  Sum/1 -> Sample and Hold_3/1
  Product1/1 -> MinMax1/1, Sum1/1, Pulse_counter_sampler (1-6)/1(angles(1-6))  "gamma(1_6)"
  Edge Detector_2/1 -> Sample and Hold_2/2, Sample and Hold_3/2, Zero crossing interpolation/2(Sample)
  Pulses(1-6)/1 -> Pulse_counter_sampler (1-6)/Trigger, Logical Operator2/1
  Logical Operator2/1 -> Logical Operator1/2
  I_th(1-6)/1 -> Hit (Falling)/1
  Logical Operator1/1 -> Monostable_1 (4 deg)/1
  Hit (Falling)/1 -> Logical Operator1/1
  Constant/1 -> Zero crossing interpolation/Enable, Divide1/1
  Clock/1 -> Sample and Hold_2/1, Sample and Hold_1/1
  Zero crossing interpolation/1(t_err) -> Divide1/2  "correction"
  Bistable/1 -> Edge Detector_1/1
  Monostable_2 (86 deg)/1 -> Bistable/2
  Bistable/2 -> Edge Detector_2/1
  Edge Detector_1/1 -> Sample and Hold_1/2
  Sample and Hold_2/1 -> Subtract1/1  "t1_tmp"

== system power_hvdc12_fault/Inverter Control and Protection/Inverter Pole Control (Current//Voltage//Gamma)/Alpha Control ==
  note: Alpha Control
  Forced_alpha : Inport
  D_alpha : Inport  Port=2
  Constant1 : Constant  Value=alpha_min
  Constant2 : Constant  Value=alpha_max
  Constant3 : Constant  Value=test_alpha
  Data Type Conversion : DataTypeConversion  OutDataTypeStr=boolean  SaturateOnIntegerOverflow=on  RndMeth=Zero
  Logical Operator : Logic  Operator=OR
  "Rate Limiter (Rate limit) " : RateLimiter  RisingSlewLimit=PRate_fix  FallingSlewLimit=NRate_fix
  "Rate Limiter (Rate limit)    " : RateLimiter  RisingSlewLimit=PRate_fix  FallingSlewLimit=NRate_fix
  Sum : Sum  Inputs=-+  SaturateOnIntegerOverflow=on  InputSameDT=on  OutDataTypeStr=Inherit: Same as first input
  Switch : Switch  Criteria=u2 > Threshold  SaturateOnIntegerOverflow=on  InputSameDT=on
  Switch1 : Switch  Criteria=u2 > Threshold  SaturateOnIntegerOverflow=on  InputSameDT=on
  fixed alpha (deg) : Constant  Value=alpha_fix
  Max_i : Outport
  Min_i : Outport  Port=2
  wires:
  "Rate Limiter (Rate limit)    "/1 -> Min_i/1
  "Rate Limiter (Rate limit) "/1 -> Max_i/1
  D_alpha/1 -> Sum/1
  Sum/1 -> Switch/3
  Constant2/1 -> Sum/2
  Constant3/1 -> Logical Operator/1
  Logical Operator/1 -> Switch/2, Switch1/2
  Constant1/1 -> Switch1/3
  Switch/1 -> "Rate Limiter (Rate limit) "/1
  Switch1/1 -> "Rate Limiter (Rate limit)    "/1
  fixed alpha (deg)/1 -> Switch/1, Switch1/1
  Forced_alpha/1 -> Data Type Conversion/1
  Data Type Conversion/1 -> Logical Operator/2
